simulink model "CDPR_bloques_lazo_abiertoR2020a"  (R2020a)
settings: Solver=ode15s  StartTime=0.0  StopTime=10  MaxStep=0.001  RelTol=1e-30
InitFcn:
  | % The global parameters for simulink are defined by running this script
  | % - Back emf constant           [Kb] (V/rad/sec)
  | % - Motor torque constant       [Kt] (N.m/A)
  | % - Mechanical inertia          [Jm] (kg.m^2)
  | % - Friction coeficient         [Bm] (N.m.s)
  | % - Armature resistance         [Ra] (Ohm)
  | % - Armature inductance         [La] (H)
  | 
  | Kb = 1.25;
  | Kt = 0.516;
  | Jm = 0.0221;
  | Bm = 0.002953;
  | Ra = 2.581;
  | La = 0.0281;
  | b = 0.1;
  | m = 0.5;
  | g = 9.81;
  | r = 0.3;
settings Model: OrderedModelArguments=off  Creator=C20256  LastModifiedBy=C20256
settings DebuggingCC: AlgebraicLoopMsg=none

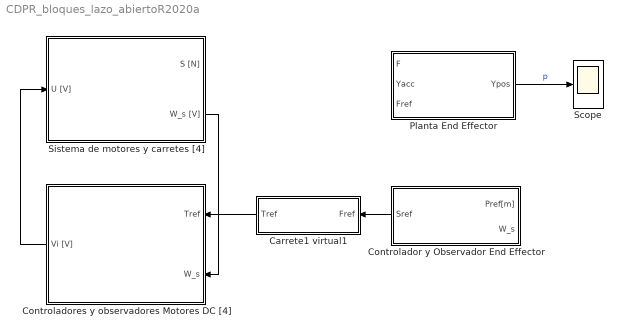
== system CDPR_bloques_lazo_abiertoR2020a ==
  Carrete1 virtual1 : Subsystem
      settings: PortSchema="{\"entries\":[{\"content\":{\"sides\":[{\"content\":{\"connectorIds\":[\"Out1\"]},\"type\":\"ConnectorPlacement.EquallySpacedRectSide\",\"uuid\":\"e435b17b-c2fe-4911-bfed-03351310c969\"},{\"content\":{\"connectorIds\":[\"In1\"],\"side\":\"RIGHT\"},\"type\":\"ConnectorPlacement.EquallySpacedRectSide\",\"uuid\":\"de4daf8e-4374-4970-b69a-ffc749c87b1a\"},{\"content\":{\"connectorIds\":[],\"side\":\"TOP\"},\"type\":\"ConnectorPlacement.EquallySpacedRectSide\",\"uuid\":\"7861d55a-b03c-4daa-b9ee-ff2ad3262c5d\"}]},\"type\":\"ConnectorPlacement.EquallySpacedConnector\",\"uuid\":\"ff68927d-1fa0-407f-8d33-41a83477036e\"}],\"packageUris\":[\"http://schema.mathworks.com/mf0/Connector/19700101\"],\"version\":\"1.0\"}"
  Controlador y Observador End Effector : Subsystem
      settings: PortSchema="{\"entries\":[{\"content\":{\"sides\":[{\"content\":{\"connectorIds\":[\"Out1\"]},\"type\":\"ConnectorPlacement.EquallySpacedRectSide\",\"uuid\":\"e435b17b-c2fe-4911-bfed-03351310c969\"},{\"content\":{\"connectorIds\":[\"In1\",\"In2\"],\"side\":\"RIGHT\"},\"type\":\"ConnectorPlacement.EquallySpacedRectSide\",\"uuid\":\"de4daf8e-4374-4970-b69a-ffc749c87b1a\"},{\"content\":{\"connectorIds\":[],\"side\":\"TOP\"},\"type\":\"ConnectorPlacement.EquallySpacedRectSide\",\"uuid\":\"7861d55a-b03c-4daa-b9ee-ff2ad3262c5d\"}]},\"type\":\"ConnectorPlacement.EquallySpacedConnector\",\"uuid\":\"ff68927d-1fa0-407f-8d33-41a83477036e\"}],\"packageUris\":[\"http://schema.mathworks.com/mf0/Connector/19700101\"],\"version\":\"1.0\"}"
  "Controladores y observadores Motores DC [4] " : Subsystem
  Planta End Effector : Subsystem
      settings: PortSchema="{\"entries\":[{\"content\":{\"sides\":[{\"content\":{\"connectorIds\":[\"In1\",\"Out2\",\"Out3\"]},\"type\":\"ConnectorPlacement.EquallySpacedRectSide\",\"uuid\":\"e435b17b-c2fe-4911-bfed-03351310c969\"},{\"content\":{\"connectorIds\":[\"Out1\"],\"side\":\"RIGHT\"},\"type\":\"ConnectorPlacement.EquallySpacedRectSide\",\"uuid\":\"de4daf8e-4374-4970-b69a-ffc749c87b1a\"},{\"content\":{\"connectorIds\":[],\"side\":\"TOP\"},\"type\":\"ConnectorPlacement.EquallySpacedRectSide\",\"uuid\":\"7861d55a-b03c-4daa-b9ee-ff2ad3262c5d\"}]},\"type\":\"ConnectorPlacement.EquallySpacedConnector\",\"uuid\":\"ff68927d-1fa0-407f-8d33-41a83477036e\"}],\"packageUris\":[\"http://schema.mathworks.com/mf0/Connector/19700101\"],\"version\":\"1.0\"}"
  Scope : Scope
  Sistema de motores y carretes [4] : Subsystem
  wires:
  Planta End Effector/1(Ypos) -> Scope/1  "p"
  "Controladores y observadores Motores DC [4] "/1(Vi [V]) -> Sistema de motores y carretes [4]/1(U [V])
  Sistema de motores y carretes [4]/2(W_s [V]) -> "Controladores y observadores Motores DC [4] "/2(W_s)
  Carrete1 virtual1/1(Tref) -> "Controladores y observadores Motores DC [4] "/1(Tref)
  Controlador y Observador End Effector/1(Sref) -> Carrete1 virtual1/1(Fref)

== system CDPR_bloques_lazo_abiertoR2020a/Carrete1 virtual1 ==
  Fref : Inport
  Gain2 : Gain  Gain=0.05
  Tref : Outport
  wires:
  Fref/1 -> Gain2/1  "Fref"
  Gain2/1 -> Tref/1  "Tref"

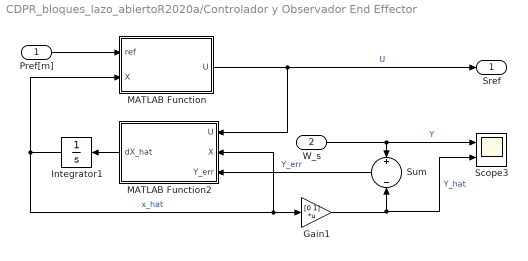
== system CDPR_bloques_lazo_abiertoR2020a/Controlador y Observador End Effector ==
  Pref[m] : Inport
  W_s : Inport  Port=2
  Gain1 : Gain  Gain=[0 1]  Multiplication=Matrix(K*u)
  Integrator1 : Integrator  InitialCondition=[0 0]
  MATLAB Function : MATLAB Function  TreatAsAtomicUnit=on
  MATLAB Function2 : MATLAB Function  TreatAsAtomicUnit=on
  Scope3 : Scope  NumInputPorts=2
  Sum : Sum  Inputs=+||||-
  Sref : Outport
  wires:
  Integrator1/1 -> MATLAB Function/2(X), Gain1/1, MATLAB Function2/2(X)  "x_hat"
  MATLAB Function2/1(dX_hat) -> Integrator1/1
  Sum/1 -> MATLAB Function2/3(Y_err)  "Y_err"
  Pref[m]/1 -> MATLAB Function/1(ref)
  Gain1/1 -> Scope3/2, Sum/2  "Y_hat"
  W_s/1 -> Scope3/1, Sum/1  "Y"
  MATLAB Function/1(U) -> Sref/1, MATLAB Function2/1(U)  "U"

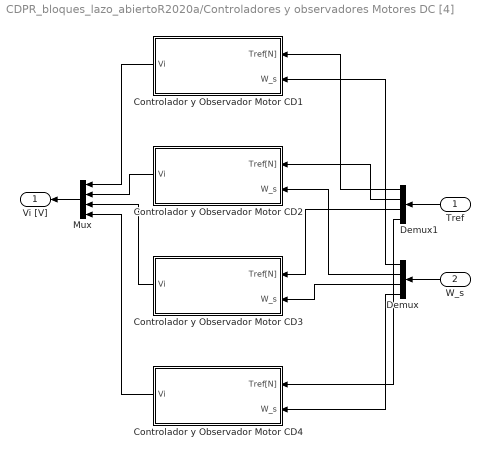
== system CDPR_bloques_lazo_abiertoR2020a/Controladores y observadores Motores DC [4]  ==
  Tref : Inport
  W_s : Inport  Port=2
  Controlador y Observador Motor CD1 : Subsystem
      settings: PortSchema="{\"entries\":[{\"content\":{\"sides\":[{\"content\":{\"connectorIds\":[\"Out1\"]},\"type\":\"ConnectorPlacement.EquallySpacedRectSide\",\"uuid\":\"e435b17b-c2fe-4911-bfed-03351310c969\"},{\"content\":{\"connectorIds\":[\"In1\",\"In2\"],\"side\":\"RIGHT\"},\"type\":\"ConnectorPlacement.EquallySpacedRectSide\",\"uuid\":\"de4daf8e-4374-4970-b69a-ffc749c87b1a\"},{\"content\":{\"connectorIds\":[],\"side\":\"TOP\"},\"type\":\"ConnectorPlacement.EquallySpacedRectSide\",\"uuid\":\"7861d55a-b03c-4daa-b9ee-ff2ad3262c5d\"}]},\"type\":\"ConnectorPlacement.EquallySpacedConnector\",\"uuid\":\"ff68927d-1fa0-407f-8d33-41a83477036e\"}],\"packageUris\":[\"http://schema.mathworks.com/mf0/Connector/19700101\"],\"version\":\"1.0\"}"
  Controlador y Observador Motor CD2 : Subsystem
      settings: PortSchema="{\"entries\":[{\"content\":{\"sides\":[{\"content\":{\"connectorIds\":[\"Out1\"]},\"type\":\"ConnectorPlacement.EquallySpacedRectSide\",\"uuid\":\"e435b17b-c2fe-4911-bfed-03351310c969\"},{\"content\":{\"connectorIds\":[\"In1\",\"In2\"],\"side\":\"RIGHT\"},\"type\":\"ConnectorPlacement.EquallySpacedRectSide\",\"uuid\":\"de4daf8e-4374-4970-b69a-ffc749c87b1a\"},{\"content\":{\"connectorIds\":[],\"side\":\"TOP\"},\"type\":\"ConnectorPlacement.EquallySpacedRectSide\",\"uuid\":\"7861d55a-b03c-4daa-b9ee-ff2ad3262c5d\"}]},\"type\":\"ConnectorPlacement.EquallySpacedConnector\",\"uuid\":\"ff68927d-1fa0-407f-8d33-41a83477036e\"}],\"packageUris\":[\"http://schema.mathworks.com/mf0/Connector/19700101\"],\"version\":\"1.0\"}"
  Controlador y Observador Motor CD3 : Subsystem
      settings: PortSchema="{\"entries\":[{\"content\":{\"sides\":[{\"content\":{\"connectorIds\":[\"Out1\"]},\"type\":\"ConnectorPlacement.EquallySpacedRectSide\",\"uuid\":\"e435b17b-c2fe-4911-bfed-03351310c969\"},{\"content\":{\"connectorIds\":[\"In1\",\"In2\"],\"side\":\"RIGHT\"},\"type\":\"ConnectorPlacement.EquallySpacedRectSide\",\"uuid\":\"de4daf8e-4374-4970-b69a-ffc749c87b1a\"},{\"content\":{\"connectorIds\":[],\"side\":\"TOP\"},\"type\":\"ConnectorPlacement.EquallySpacedRectSide\",\"uuid\":\"7861d55a-b03c-4daa-b9ee-ff2ad3262c5d\"}]},\"type\":\"ConnectorPlacement.EquallySpacedConnector\",\"uuid\":\"ff68927d-1fa0-407f-8d33-41a83477036e\"}],\"packageUris\":[\"http://schema.mathworks.com/mf0/Connector/19700101\"],\"version\":\"1.0\"}"
  Controlador y Observador Motor CD4 : Subsystem
      settings: PortSchema="{\"entries\":[{\"content\":{\"sides\":[{\"content\":{\"connectorIds\":[\"Out1\"]},\"type\":\"ConnectorPlacement.EquallySpacedRectSide\",\"uuid\":\"e435b17b-c2fe-4911-bfed-03351310c969\"},{\"content\":{\"connectorIds\":[\"In1\",\"In2\"],\"side\":\"RIGHT\"},\"type\":\"ConnectorPlacement.EquallySpacedRectSide\",\"uuid\":\"de4daf8e-4374-4970-b69a-ffc749c87b1a\"},{\"content\":{\"connectorIds\":[],\"side\":\"TOP\"},\"type\":\"ConnectorPlacement.EquallySpacedRectSide\",\"uuid\":\"7861d55a-b03c-4daa-b9ee-ff2ad3262c5d\"}]},\"type\":\"ConnectorPlacement.EquallySpacedConnector\",\"uuid\":\"ff68927d-1fa0-407f-8d33-41a83477036e\"}],\"packageUris\":[\"http://schema.mathworks.com/mf0/Connector/19700101\"],\"version\":\"1.0\"}"
  Demux : Demux
  Demux1 : Demux
  Mux : Mux
  Vi [V] : Outport
  wires:
  W_s/1 -> Demux/1
  Tref/1 -> Demux1/1
  Demux1/1 -> Controlador y Observador Motor CD1/1(Tref[N])
  Demux1/2 -> Controlador y Observador Motor CD2/1(Tref[N])
  Demux1/3 -> Controlador y Observador Motor CD3/1(Tref[N])
  Demux1/4 -> Controlador y Observador Motor CD4/1(Tref[N])
  Demux/1 -> Controlador y Observador Motor CD1/2(W_s)
  Demux/2 -> Controlador y Observador Motor CD2/2(W_s)
  Demux/3 -> Controlador y Observador Motor CD3/2(W_s)
  Demux/4 -> Controlador y Observador Motor CD4/2(W_s)
  Controlador y Observador Motor CD4/1(Vi) -> Mux/4
  Controlador y Observador Motor CD3/1(Vi) -> Mux/3
  Mux/1 -> Vi [V]/1
  Controlador y Observador Motor CD2/1(Vi) -> Mux/2
  Controlador y Observador Motor CD1/1(Vi) -> Mux/1

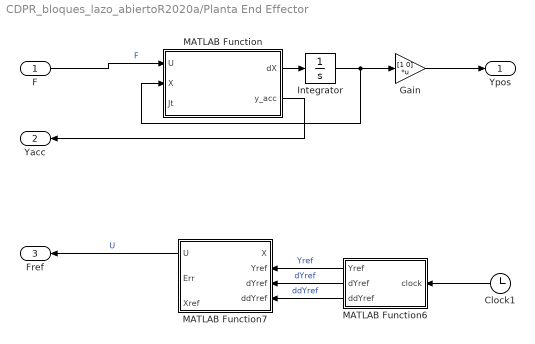
== system CDPR_bloques_lazo_abiertoR2020a/Planta End Effector ==
  F : Inport
  Clock1 : Clock
  Gain : Gain  Gain=[1 0]  Multiplication=Matrix(K*u)
  Integrator : Integrator  InitialCondition=[0 0]
  MATLAB Function : MATLAB Function  TreatAsAtomicUnit=on
  MATLAB Function6 : MATLAB Function  TreatAsAtomicUnit=on
  MATLAB Function7 : MATLAB Function  TreatAsAtomicUnit=on
  Ypos : Outport
  Yacc : Outport  Port=2
  Fref : Outport  Port=3
  wires:
  Integrator/1 -> Gain/1, MATLAB Function/2(X)
  MATLAB Function/1(dX) -> Integrator/1
  Gain/1 -> Ypos/1
  MATLAB Function/2(y_acc) -> Yacc/1
  Clock1/1 -> MATLAB Function6/1(clock)
  MATLAB Function6/1(Yref) -> MATLAB Function7/2(Yref)  "Yref"
  MATLAB Function6/2(dYref) -> MATLAB Function7/3(dYref)  "dYref"
  MATLAB Function6/3(ddYref) -> MATLAB Function7/4(ddYref)  "ddYref"
  MATLAB Function7/1(U) -> Fref/1  "U"
  F/1 -> MATLAB Function/1(U)  "F"

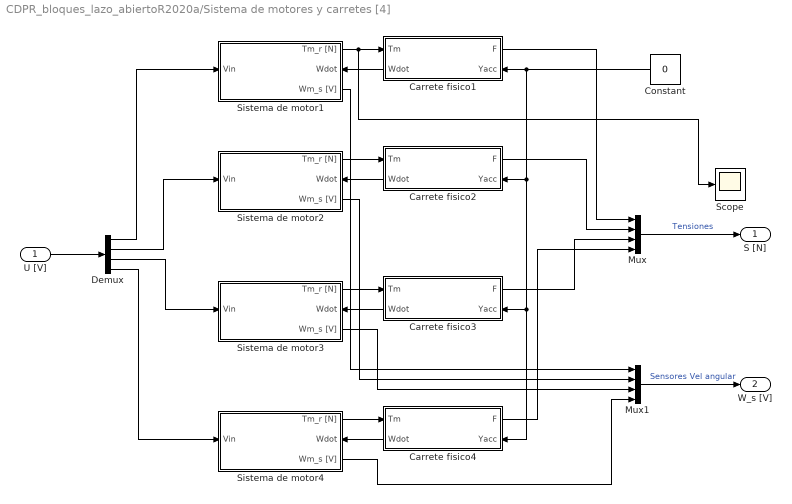
== system CDPR_bloques_lazo_abiertoR2020a/Sistema de motores y carretes [4] ==
  U [V] : Inport
  Carrete fisico1 : Subsystem
      settings: PortSchema="{\"entries\":[{\"content\":{\"sides\":[{\"content\":{\"connectorIds\":[\"In1\",\"Out2\"]},\"type\":\"ConnectorPlacement.EquallySpacedRectSide\",\"uuid\":\"e435b17b-c2fe-4911-bfed-03351310c969\"},{\"content\":{\"connectorIds\":[\"Out1\",\"In2\"],\"side\":\"RIGHT\"},\"type\":\"ConnectorPlacement.EquallySpacedRectSide\",\"uuid\":\"de4daf8e-4374-4970-b69a-ffc749c87b1a\"},{\"content\":{\"connectorIds\":[],\"side\":\"TOP\"},\"type\":\"ConnectorPlacement.EquallySpacedRectSide\",\"uuid\":\"7861d55a-b03c-4daa-b9ee-ff2ad3262c5d\"}]},\"type\":\"ConnectorPlacement.EquallySpacedConnector\",\"uuid\":\"ff68927d-1fa0-407f-8d33-41a83477036e\"}],\"packageUris\":[\"http://schema.mathworks.com/mf0/Connector/19700101\"],\"version\":\"1.0\"}"
  Carrete fisico2 : Subsystem
      settings: PortSchema="{\"entries\":[{\"content\":{\"sides\":[{\"content\":{\"connectorIds\":[\"In1\",\"Out2\"]},\"type\":\"ConnectorPlacement.EquallySpacedRectSide\",\"uuid\":\"e435b17b-c2fe-4911-bfed-03351310c969\"},{\"content\":{\"connectorIds\":[\"Out1\",\"In2\"],\"side\":\"RIGHT\"},\"type\":\"ConnectorPlacement.EquallySpacedRectSide\",\"uuid\":\"de4daf8e-4374-4970-b69a-ffc749c87b1a\"},{\"content\":{\"connectorIds\":[],\"side\":\"TOP\"},\"type\":\"ConnectorPlacement.EquallySpacedRectSide\",\"uuid\":\"7861d55a-b03c-4daa-b9ee-ff2ad3262c5d\"}]},\"type\":\"ConnectorPlacement.EquallySpacedConnector\",\"uuid\":\"ff68927d-1fa0-407f-8d33-41a83477036e\"}],\"packageUris\":[\"http://schema.mathworks.com/mf0/Connector/19700101\"],\"version\":\"1.0\"}"
  Carrete fisico3 : Subsystem
      settings: PortSchema="{\"entries\":[{\"content\":{\"sides\":[{\"content\":{\"connectorIds\":[\"In1\",\"Out2\"]},\"type\":\"ConnectorPlacement.EquallySpacedRectSide\",\"uuid\":\"e435b17b-c2fe-4911-bfed-03351310c969\"},{\"content\":{\"connectorIds\":[\"Out1\",\"In2\"],\"side\":\"RIGHT\"},\"type\":\"ConnectorPlacement.EquallySpacedRectSide\",\"uuid\":\"de4daf8e-4374-4970-b69a-ffc749c87b1a\"},{\"content\":{\"connectorIds\":[],\"side\":\"TOP\"},\"type\":\"ConnectorPlacement.EquallySpacedRectSide\",\"uuid\":\"7861d55a-b03c-4daa-b9ee-ff2ad3262c5d\"}]},\"type\":\"ConnectorPlacement.EquallySpacedConnector\",\"uuid\":\"ff68927d-1fa0-407f-8d33-41a83477036e\"}],\"packageUris\":[\"http://schema.mathworks.com/mf0/Connector/19700101\"],\"version\":\"1.0\"}"
  Carrete fisico4 : Subsystem
      settings: PortSchema="{\"entries\":[{\"content\":{\"sides\":[{\"content\":{\"connectorIds\":[\"In1\",\"Out2\"]},\"type\":\"ConnectorPlacement.EquallySpacedRectSide\",\"uuid\":\"e435b17b-c2fe-4911-bfed-03351310c969\"},{\"content\":{\"connectorIds\":[\"Out1\",\"In2\"],\"side\":\"RIGHT\"},\"type\":\"ConnectorPlacement.EquallySpacedRectSide\",\"uuid\":\"de4daf8e-4374-4970-b69a-ffc749c87b1a\"},{\"content\":{\"connectorIds\":[],\"side\":\"TOP\"},\"type\":\"ConnectorPlacement.EquallySpacedRectSide\",\"uuid\":\"7861d55a-b03c-4daa-b9ee-ff2ad3262c5d\"}]},\"type\":\"ConnectorPlacement.EquallySpacedConnector\",\"uuid\":\"ff68927d-1fa0-407f-8d33-41a83477036e\"}],\"packageUris\":[\"http://schema.mathworks.com/mf0/Connector/19700101\"],\"version\":\"1.0\"}"
  Constant : Constant  Value=0
  Demux : Demux
  Mux : Mux
  Mux1 : Mux
  Scope : Scope
  Sistema de motor1 : Subsystem
      settings: PortSchema="{\"entries\":[{\"content\":{\"sides\":[{\"content\":{\"connectorIds\":[\"In1\"]},\"type\":\"ConnectorPlacement.EquallySpacedRectSide\",\"uuid\":\"e435b17b-c2fe-4911-bfed-03351310c969\"},{\"content\":{\"connectorIds\":[\"Out1\",\"In2\",\"Out2\"],\"side\":\"RIGHT\"},\"type\":\"ConnectorPlacement.EquallySpacedRectSide\",\"uuid\":\"de4daf8e-4374-4970-b69a-ffc749c87b1a\"},{\"content\":{\"connectorIds\":[],\"side\":\"TOP\"},\"type\":\"ConnectorPlacement.EquallySpacedRectSide\",\"uuid\":\"7861d55a-b03c-4daa-b9ee-ff2ad3262c5d\"}]},\"type\":\"ConnectorPlacement.EquallySpacedConnector\",\"uuid\":\"ff68927d-1fa0-407f-8d33-41a83477036e\"}],\"packageUris\":[\"http://schema.mathworks.com/mf0/Connector/19700101\"],\"version\":\"1.0\"}"
  Sistema de motor2 : Subsystem
      settings: PortSchema="{\"entries\":[{\"content\":{\"sides\":[{\"content\":{\"connectorIds\":[\"In1\"]},\"type\":\"ConnectorPlacement.EquallySpacedRectSide\",\"uuid\":\"e435b17b-c2fe-4911-bfed-03351310c969\"},{\"content\":{\"connectorIds\":[\"Out1\",\"In2\",\"Out2\"],\"side\":\"RIGHT\"},\"type\":\"ConnectorPlacement.EquallySpacedRectSide\",\"uuid\":\"de4daf8e-4374-4970-b69a-ffc749c87b1a\"},{\"content\":{\"connectorIds\":[],\"side\":\"TOP\"},\"type\":\"ConnectorPlacement.EquallySpacedRectSide\",\"uuid\":\"7861d55a-b03c-4daa-b9ee-ff2ad3262c5d\"}]},\"type\":\"ConnectorPlacement.EquallySpacedConnector\",\"uuid\":\"ff68927d-1fa0-407f-8d33-41a83477036e\"}],\"packageUris\":[\"http://schema.mathworks.com/mf0/Connector/19700101\"],\"version\":\"1.0\"}"
  Sistema de motor3 : Subsystem
      settings: PortSchema="{\"entries\":[{\"content\":{\"sides\":[{\"content\":{\"connectorIds\":[\"In1\"]},\"type\":\"ConnectorPlacement.EquallySpacedRectSide\",\"uuid\":\"e435b17b-c2fe-4911-bfed-03351310c969\"},{\"content\":{\"connectorIds\":[\"Out1\",\"In2\",\"Out2\"],\"side\":\"RIGHT\"},\"type\":\"ConnectorPlacement.EquallySpacedRectSide\",\"uuid\":\"de4daf8e-4374-4970-b69a-ffc749c87b1a\"},{\"content\":{\"connectorIds\":[],\"side\":\"TOP\"},\"type\":\"ConnectorPlacement.EquallySpacedRectSide\",\"uuid\":\"7861d55a-b03c-4daa-b9ee-ff2ad3262c5d\"}]},\"type\":\"ConnectorPlacement.EquallySpacedConnector\",\"uuid\":\"ff68927d-1fa0-407f-8d33-41a83477036e\"}],\"packageUris\":[\"http://schema.mathworks.com/mf0/Connector/19700101\"],\"version\":\"1.0\"}"
  Sistema de motor4 : Subsystem
      settings: PortSchema="{\"entries\":[{\"content\":{\"sides\":[{\"content\":{\"connectorIds\":[\"In1\"]},\"type\":\"ConnectorPlacement.EquallySpacedRectSide\",\"uuid\":\"e435b17b-c2fe-4911-bfed-03351310c969\"},{\"content\":{\"connectorIds\":[\"Out1\",\"In2\",\"Out2\"],\"side\":\"RIGHT\"},\"type\":\"ConnectorPlacement.EquallySpacedRectSide\",\"uuid\":\"de4daf8e-4374-4970-b69a-ffc749c87b1a\"},{\"content\":{\"connectorIds\":[],\"side\":\"TOP\"},\"type\":\"ConnectorPlacement.EquallySpacedRectSide\",\"uuid\":\"7861d55a-b03c-4daa-b9ee-ff2ad3262c5d\"}]},\"type\":\"ConnectorPlacement.EquallySpacedConnector\",\"uuid\":\"ff68927d-1fa0-407f-8d33-41a83477036e\"}],\"packageUris\":[\"http://schema.mathworks.com/mf0/Connector/19700101\"],\"version\":\"1.0\"}"
  S [N] : Outport
  W_s [V] : Outport  Port=2
  wires:
  Sistema de motor3/2(Wm_s [V]) -> Mux1/3
  Carrete fisico3/2(Wdot) -> Sistema de motor3/2(Wdot)
  Sistema de motor1/2(Wm_s [V]) -> Mux1/1
  Carrete fisico2/2(Wdot) -> Sistema de motor2/2(Wdot)
  Sistema de motor3/1(Tm_r [N]) -> Carrete fisico3/1(Tm)
  Sistema de motor4/2(Wm_s [V]) -> Mux1/4
  Sistema de motor1/1(Tm_r [N]) -> Scope/1, Carrete fisico1/1(Tm)
  Sistema de motor2/2(Wm_s [V]) -> Mux1/2
  Carrete fisico4/2(Wdot) -> Sistema de motor4/2(Wdot)
  Sistema de motor2/1(Tm_r [N]) -> Carrete fisico2/1(Tm)
  Carrete fisico1/2(Wdot) -> Sistema de motor1/2(Wdot)
  Sistema de motor4/1(Tm_r [N]) -> Carrete fisico4/1(Tm)
  Demux/1 -> Sistema de motor1/1(Vin)
  Demux/2 -> Sistema de motor2/1(Vin)
  Demux/3 -> Sistema de motor3/1(Vin)
  Demux/4 -> Sistema de motor4/1(Vin)
  U [V]/1 -> Demux/1
  Carrete fisico2/1(F) -> Mux/2
  Carrete fisico1/1(F) -> Mux/1
  Carrete fisico3/1(F) -> Mux/3
  Carrete fisico4/1(F) -> Mux/4
  Mux1/1 -> W_s [V]/1  "Sensores Vel angular"
  Mux/1 -> S [N]/1  "Tensiones"
  Constant/1 -> Carrete fisico4/2(Yacc), Carrete fisico3/2(Yacc), Carrete fisico2/2(Yacc), Carrete fisico1/2(Yacc)

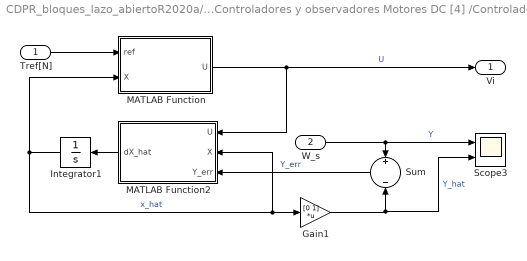
== system CDPR_bloques_lazo_abiertoR2020a/Controladores y observadores Motores DC [4] /Controlador y Observador Motor CD1 ==
  Tref[N] : Inport
  W_s : Inport  Port=2
  Gain1 : Gain  Gain=[0 1]  Multiplication=Matrix(K*u)
  Integrator1 : Integrator  InitialCondition=[0 0]
  MATLAB Function : MATLAB Function  TreatAsAtomicUnit=on
  MATLAB Function2 : MATLAB Function  TreatAsAtomicUnit=on
  Scope3 : Scope  NumInputPorts=2
  Sum : Sum  Inputs=+||||-
  Vi : Outport
  wires:
  Integrator1/1 -> MATLAB Function/2(X), Gain1/1, MATLAB Function2/2(X)  "x_hat"
  MATLAB Function2/1(dX_hat) -> Integrator1/1
  Sum/1 -> MATLAB Function2/3(Y_err)  "Y_err"
  Tref[N]/1 -> MATLAB Function/1(ref)
  Gain1/1 -> Scope3/2, Sum/2  "Y_hat"
  W_s/1 -> Scope3/1, Sum/1  "Y"
  MATLAB Function/1(U) -> Vi/1, MATLAB Function2/1(U)  "U"

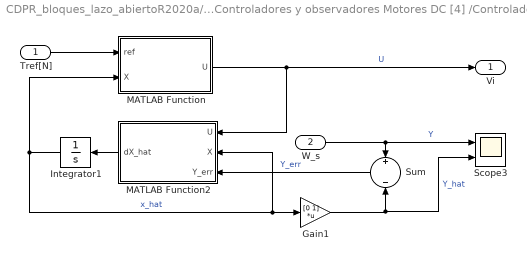
== system CDPR_bloques_lazo_abiertoR2020a/Controladores y observadores Motores DC [4] /Controlador y Observador Motor CD2 ==
  Tref[N] : Inport
  W_s : Inport  Port=2
  Gain1 : Gain  Gain=[0 1]  Multiplication=Matrix(K*u)
  Integrator1 : Integrator  InitialCondition=[0 0]
  MATLAB Function : MATLAB Function  TreatAsAtomicUnit=on
  MATLAB Function2 : MATLAB Function  TreatAsAtomicUnit=on
  Scope3 : Scope  NumInputPorts=2
  Sum : Sum  Inputs=+||||-
  Vi : Outport
  wires:
  Integrator1/1 -> MATLAB Function/2(X), Gain1/1, MATLAB Function2/2(X)  "x_hat"
  MATLAB Function2/1(dX_hat) -> Integrator1/1
  Sum/1 -> MATLAB Function2/3(Y_err)  "Y_err"
  Tref[N]/1 -> MATLAB Function/1(ref)
  Gain1/1 -> Scope3/2, Sum/2  "Y_hat"
  W_s/1 -> Scope3/1, Sum/1  "Y"
  MATLAB Function/1(U) -> Vi/1, MATLAB Function2/1(U)  "U"

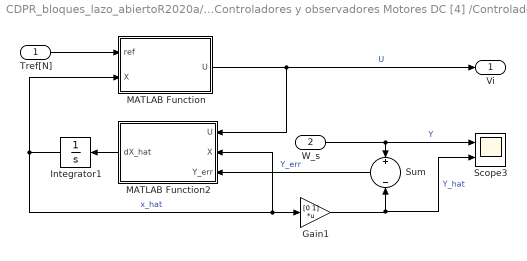
== system CDPR_bloques_lazo_abiertoR2020a/Controladores y observadores Motores DC [4] /Controlador y Observador Motor CD3 ==
  Tref[N] : Inport
  W_s : Inport  Port=2
  Gain1 : Gain  Gain=[0 1]  Multiplication=Matrix(K*u)
  Integrator1 : Integrator  InitialCondition=[0 0]
  MATLAB Function : MATLAB Function  TreatAsAtomicUnit=on
  MATLAB Function2 : MATLAB Function  TreatAsAtomicUnit=on
  Scope3 : Scope  NumInputPorts=2
  Sum : Sum  Inputs=+||||-
  Vi : Outport
  wires:
  Integrator1/1 -> MATLAB Function/2(X), Gain1/1, MATLAB Function2/2(X)  "x_hat"
  MATLAB Function2/1(dX_hat) -> Integrator1/1
  Sum/1 -> MATLAB Function2/3(Y_err)  "Y_err"
  Tref[N]/1 -> MATLAB Function/1(ref)
  Gain1/1 -> Scope3/2, Sum/2  "Y_hat"
  W_s/1 -> Scope3/1, Sum/1  "Y"
  MATLAB Function/1(U) -> Vi/1, MATLAB Function2/1(U)  "U"

== system CDPR_bloques_lazo_abiertoR2020a/Controladores y observadores Motores DC [4] /Controlador y Observador Motor CD4 ==
  Tref[N] : Inport
  W_s : Inport  Port=2
  Gain1 : Gain  Gain=[0 1]  Multiplication=Matrix(K*u)
  Integrator1 : Integrator  InitialCondition=[0 0]
  MATLAB Function : MATLAB Function  TreatAsAtomicUnit=on
  MATLAB Function2 : MATLAB Function  TreatAsAtomicUnit=on
  Scope3 : Scope  NumInputPorts=2
  Sum : Sum  Inputs=+||||-
  Vi : Outport
  wires:
  Integrator1/1 -> MATLAB Function/2(X), Gain1/1, MATLAB Function2/2(X)  "x_hat"
  MATLAB Function2/1(dX_hat) -> Integrator1/1
  Sum/1 -> MATLAB Function2/3(Y_err)  "Y_err"
  Tref[N]/1 -> MATLAB Function/1(ref)
  Gain1/1 -> Scope3/2, Sum/2  "Y_hat"
  W_s/1 -> Scope3/1, Sum/1  "Y"
  MATLAB Function/1(U) -> Vi/1, MATLAB Function2/1(U)  "U"

== system CDPR_bloques_lazo_abiertoR2020a/Sistema de motores y carretes [4]/Carrete fisico1 ==
  Tm : Inport
  Yacc : Inport  Port=2
  Gain : Gain  Gain=1/0.05
  Gain1 : Gain  Gain=1/0.05
  F : Outport
  Wdot : Outport  Port=2
  wires:
  Tm/1 -> Gain/1  "Tm"
  Gain/1 -> F/1  "F"
  Yacc/1 -> Gain1/1  "Yacc"
  Gain1/1 -> Wdot/1  "Acc ang"

== system CDPR_bloques_lazo_abiertoR2020a/Sistema de motores y carretes [4]/Carrete fisico2 ==
  Tm : Inport
  Yacc : Inport  Port=2
  Gain : Gain  Gain=1/0.05
  Gain1 : Gain  Gain=1/0.05
  F : Outport
  Wdot : Outport  Port=2
  wires:
  Tm/1 -> Gain/1  "Tm"
  Gain/1 -> F/1  "F"
  Yacc/1 -> Gain1/1  "Yacc"
  Gain1/1 -> Wdot/1  "Acc ang"

== system CDPR_bloques_lazo_abiertoR2020a/Sistema de motores y carretes [4]/Carrete fisico3 ==
  Tm : Inport
  Yacc : Inport  Port=2
  Gain : Gain  Gain=1/0.05
  Gain1 : Gain  Gain=1/0.05
  F : Outport
  Wdot : Outport  Port=2
  wires:
  Tm/1 -> Gain/1  "Tm"
  Gain/1 -> F/1  "F"
  Yacc/1 -> Gain1/1  "Yacc"
  Gain1/1 -> Wdot/1  "Acc ang"

== system CDPR_bloques_lazo_abiertoR2020a/Sistema de motores y carretes [4]/Carrete fisico4 ==
  Tm : Inport
  Yacc : Inport  Port=2
  Gain : Gain  Gain=1/0.05
  Gain1 : Gain  Gain=1/0.05
  F : Outport
  Wdot : Outport  Port=2
  wires:
  Tm/1 -> Gain/1  "Tm"
  Gain/1 -> F/1  "F"
  Yacc/1 -> Gain1/1  "Yacc"
  Gain1/1 -> Wdot/1  "Acc ang"

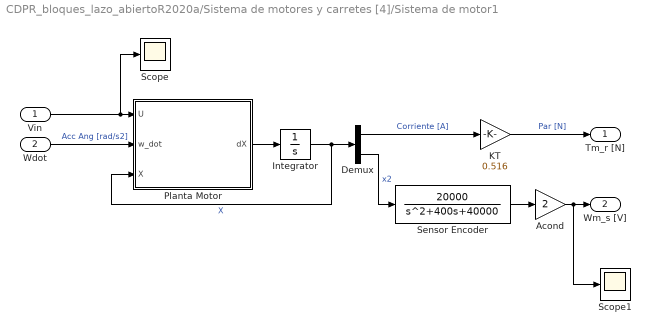
== system CDPR_bloques_lazo_abiertoR2020a/Sistema de motores y carretes [4]/Sistema de motor1 ==
  Vin : Inport
  Wdot : Inport  Port=2
  Acond : Gain  Gain=2
  Demux : Demux  Outputs=2
  Integrator : Integrator  InitialCondition=[0 0]
  KT : Gain  Gain=0.516
  Planta Motor : MATLAB Function  TreatAsAtomicUnit=on
  Scope : Scope
  Scope1 : Scope
  Sensor Encoder : TransferFcn  Numerator=[20000]  Denominator=[1 400 40000]
  Tm_r [N] : Outport
  Wm_s [V] : Outport  Port=2
  wires:
  Planta Motor/1(dX) -> Integrator/1
  Integrator/1 -> Planta Motor/3(X), Demux/1  "X"
  KT/1 -> Tm_r [N]/1  "Par [N]"
  Demux/1 -> KT/1  "Corriente [A]"
  Acond/1 -> Scope1/1, Wm_s [V]/1
  Sensor Encoder/1 -> Acond/1
  Demux/2 -> Sensor Encoder/1  "x2"
  Wdot/1 -> Planta Motor/2(w_dot)  "Acc Ang [rad/s2]"
  Vin/1 -> Scope/1, Planta Motor/1(U)

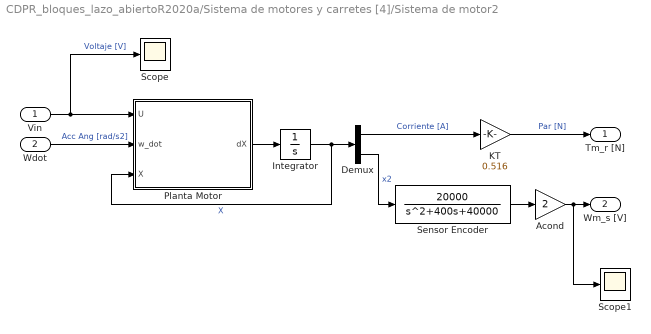
== system CDPR_bloques_lazo_abiertoR2020a/Sistema de motores y carretes [4]/Sistema de motor2 ==
  Vin : Inport
  Wdot : Inport  Port=2
  Acond : Gain  Gain=2
  Demux : Demux  Outputs=2
  Integrator : Integrator  InitialCondition=[0 0]
  KT : Gain  Gain=0.516
  Planta Motor : MATLAB Function  TreatAsAtomicUnit=on
  Scope : Scope
  Scope1 : Scope
  Sensor Encoder : TransferFcn  Numerator=[20000]  Denominator=[1 400 40000]
  Tm_r [N] : Outport
  Wm_s [V] : Outport  Port=2
  wires:
  Planta Motor/1(dX) -> Integrator/1
  Integrator/1 -> Planta Motor/3(X), Demux/1  "X"
  KT/1 -> Tm_r [N]/1  "Par [N]"
  Demux/1 -> KT/1  "Corriente [A]"
  Wdot/1 -> Planta Motor/2(w_dot)  "Acc Ang [rad/s2]"
  Vin/1 -> Scope/1, Planta Motor/1(U)  "Voltaje [V]"
  Acond/1 -> Scope1/1, Wm_s [V]/1
  Sensor Encoder/1 -> Acond/1
  Demux/2 -> Sensor Encoder/1  "x2"

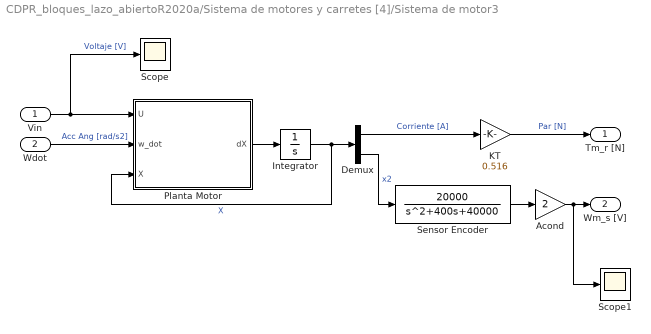
== system CDPR_bloques_lazo_abiertoR2020a/Sistema de motores y carretes [4]/Sistema de motor3 ==
  Vin : Inport
  Wdot : Inport  Port=2
  Acond : Gain  Gain=2
  Demux : Demux  Outputs=2
  Integrator : Integrator  InitialCondition=[0 0]
  KT : Gain  Gain=0.516
  Planta Motor : MATLAB Function  TreatAsAtomicUnit=on
  Scope : Scope
  Scope1 : Scope
  Sensor Encoder : TransferFcn  Numerator=[20000]  Denominator=[1 400 40000]
  Tm_r [N] : Outport
  Wm_s [V] : Outport  Port=2
  wires:
  Planta Motor/1(dX) -> Integrator/1
  Integrator/1 -> Planta Motor/3(X), Demux/1  "X"
  KT/1 -> Tm_r [N]/1  "Par [N]"
  Demux/1 -> KT/1  "Corriente [A]"
  Wdot/1 -> Planta Motor/2(w_dot)  "Acc Ang [rad/s2]"
  Vin/1 -> Scope/1, Planta Motor/1(U)  "Voltaje [V]"
  Acond/1 -> Scope1/1, Wm_s [V]/1
  Sensor Encoder/1 -> Acond/1
  Demux/2 -> Sensor Encoder/1  "x2"

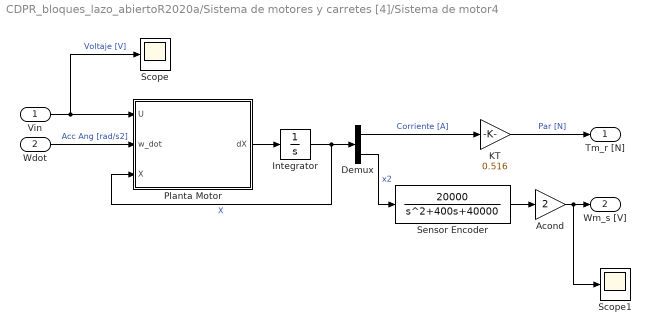
== system CDPR_bloques_lazo_abiertoR2020a/Sistema de motores y carretes [4]/Sistema de motor4 ==
  Vin : Inport
  Wdot : Inport  Port=2
  Acond : Gain  Gain=2
  Demux : Demux  Outputs=2
  Integrator : Integrator  InitialCondition=[0 0]
  KT : Gain  Gain=0.516
  Planta Motor : MATLAB Function  TreatAsAtomicUnit=on
  Scope : Scope
  Scope1 : Scope
  Sensor Encoder : TransferFcn  Numerator=[20000]  Denominator=[1 400 40000]
  Tm_r [N] : Outport
  Wm_s [V] : Outport  Port=2
  wires:
  Planta Motor/1(dX) -> Integrator/1
  Integrator/1 -> Planta Motor/3(X), Demux/1  "X"
  KT/1 -> Tm_r [N]/1  "Par [N]"
  Demux/1 -> KT/1  "Corriente [A]"
  Wdot/1 -> Planta Motor/2(w_dot)  "Acc Ang [rad/s2]"
  Vin/1 -> Scope/1, Planta Motor/1(U)  "Voltaje [V]"
  Acond/1 -> Scope1/1, Wm_s [V]/1
  Sensor Encoder/1 -> Acond/1
  Demux/2 -> Sensor Encoder/1  "x2"

== matlab function CDPR_bloques_lazo_abiertoR2020a/Sistema de motores y carretes [4]/Sistema de motor4/Planta Motor ==
  data: U input; w_dot input; dX output; X input
function dX  = MotorCD(U, w_dot, X)
%Parametros del sistema

Kb = 1.25;
Kt = 0.516;
Jm = 0.0221;
Bm = 0.002953;
Ra = 2.581;
La = 0.0281;

a11 = -Ra/La;
a12 = -Kb/La;
a21 =  Kt/Jm;
a22 = -Bm/Jm;
b11 = 1/La;
b22 = 0;
f11 = 0;
f22 = -1/Jm;
 
A = [a11 a12; a21 a22]; 
B = [b11; b22];

F = [f11; f22];
TL = -Kt * X(1) + Jm * w_dot + Bm * X(2) ;
 
dX = A*X + B*U + F*TL;
end

== matlab function CDPR_bloques_lazo_abiertoR2020a/Controladores y observadores Motores DC [4] /Controlador y Observador Motor CD2/MATLAB Function ==
  settings: updateMethod=CONTINUOUS
  data: ref input; X input; U output
function U  = Controlador(ref, X)
Kb = 1.25;
Kt = 0.516;
Jm = 0.0221;
Bm = 0.002953;
Ra = 2.581;
La = 0.0281;

a11 = -Ra/La;
a12 = -Kb/La;
a21 =  Kt/Jm;
a22 = -Bm/Jm;
b11 = 1/La;
b22 = 0;
 
A = [a11 a12; a21 a22]; 
B = [b11; b22];
C = [Kt 0];
Pd = [-4 -4];
%Controlador
Mc = [B A*B]
H = (A-Pd(1)*eye(2))*(A-Pd(2)*eye(2));
K = -[0 1] * inv(Mc) * H;
F = 1/(C*inv(-A-B*K) * B);

U = K*X + F*ref;
end

== matlab function CDPR_bloques_lazo_abiertoR2020a/Controladores y observadores Motores DC [4] /Controlador y Observador Motor CD2/MATLAB Function2 ==
  data: U input; X input; Y_err input; dX_hat output
function dX_hat = Observador(U, X, Y_err)
Kb = 1.25;
Kt = 0.516;
Jm = 0.0221;
Bm = 0.002953;
Ra = 2.581;
La = 0.0281;

a11 = -Ra/La;
a12 = -Kb/La;
a21 =  Kt/Jm;
a22 = -Bm/Jm;
b11 = 1/La;
b22 = 0;
 
A = [a11 a12; a21 a22]; 
B = [b11; b22];
C = [0 1];

Pdo = [-80 -80];

Mo1 = [C ;
      C*A];
Ho = (A-Pdo(1)*eye(2))*(A-Pdo(2)*eye(2));
L = -Ho * inv(Mo1) * [0 1].';
%Espacio de estados
dX_hat = A*X + B*U - L*Y_err;
end

== matlab function CDPR_bloques_lazo_abiertoR2020a/Controladores y observadores Motores DC [4] /Controlador y Observador Motor CD3/MATLAB Function ==
  settings: updateMethod=CONTINUOUS
  data: ref input; X input; U output
function U  = Controlador(ref, X)
Kb = 1.25;
Kt = 0.516;
Jm = 0.0221;
Bm = 0.002953;
Ra = 2.581;
La = 0.0281;

a11 = -Ra/La;
a12 = -Kb/La;
a21 =  Kt/Jm;
a22 = -Bm/Jm;
b11 = 1/La;
b22 = 0;
 
A = [a11 a12; a21 a22]; 
B = [b11; b22];
C = [Kt 0];
Pd = [-4 -4];
%Controlador
Mc = [B A*B]
H = (A-Pd(1)*eye(2))*(A-Pd(2)*eye(2));
K = -[0 1] * inv(Mc) * H;
F = 1/(C*inv(-A-B*K) * B);

U = K*X + F*ref;
end

== matlab function CDPR_bloques_lazo_abiertoR2020a/Controladores y observadores Motores DC [4] /Controlador y Observador Motor CD3/MATLAB Function2 ==
  data: U input; X input; Y_err input; dX_hat output
function dX_hat = Observador(U, X, Y_err)
Kb = 1.25;
Kt = 0.516;
Jm = 0.0221;
Bm = 0.002953;
Ra = 2.581;
La = 0.0281;

a11 = -Ra/La;
a12 = -Kb/La;
a21 =  Kt/Jm;
a22 = -Bm/Jm;
b11 = 1/La;
b22 = 0;
 
A = [a11 a12; a21 a22]; 
B = [b11; b22];
C = [0 1];

Pdo = [-80 -80];

Mo1 = [C ;
      C*A];
Ho = (A-Pdo(1)*eye(2))*(A-Pdo(2)*eye(2));
L = -Ho * inv(Mo1) * [0 1].';
%Espacio de estados
dX_hat = A*X + B*U - L*Y_err;
end

== matlab function CDPR_bloques_lazo_abiertoR2020a/Controladores y observadores Motores DC [4] /Controlador y Observador Motor CD4/MATLAB Function ==
  settings: updateMethod=CONTINUOUS
  data: ref input; X input; U output
function U  = Controlador(ref, X)
Kb = 1.25;
Kt = 0.516;
Jm = 0.0221;
Bm = 0.002953;
Ra = 2.581;
La = 0.0281;

a11 = -Ra/La;
a12 = -Kb/La;
a21 =  Kt/Jm;
a22 = -Bm/Jm;
b11 = 1/La;
b22 = 0;
 
A = [a11 a12; a21 a22]; 
B = [b11; b22];
C = [Kt 0];
Pd = [-4 -4];
%Controlador
Mc = [B A*B]
H = (A-Pd(1)*eye(2))*(A-Pd(2)*eye(2));
K = -[0 1] * inv(Mc) * H;
F = 1/(C*inv(-A-B*K) * B);

U = K*X + F*ref;
end

== matlab function CDPR_bloques_lazo_abiertoR2020a/Controladores y observadores Motores DC [4] /Controlador y Observador Motor CD4/MATLAB Function2 ==
  data: U input; X input; Y_err input; dX_hat output
function dX_hat = Observador(U, X, Y_err)
Kb = 1.25;
Kt = 0.516;
Jm = 0.0221;
Bm = 0.002953;
Ra = 2.581;
La = 0.0281;

a11 = -Ra/La;
a12 = -Kb/La;
a21 =  Kt/Jm;
a22 = -Bm/Jm;
b11 = 1/La;
b22 = 0;
 
A = [a11 a12; a21 a22]; 
B = [b11; b22];
C = [0 1];

Pdo = [-80 -80];

Mo1 = [C ;
      C*A];
Ho = (A-Pdo(1)*eye(2))*(A-Pdo(2)*eye(2));
L = -Ho * inv(Mo1) * [0 1].';
%Espacio de estados
dX_hat = A*X + B*U - L*Y_err;
end

== matlab function CDPR_bloques_lazo_abiertoR2020a/Controlador y Observador End Effector/MATLAB Function ==
  settings: updateMethod=CONTINUOUS
  data: ref input; X input; U output
function U  = Controlador(ref, X)
Kb = 1.25;
Kt = 0.516;
Jm = 0.0221;
Bm = 0.002953;
Ra = 2.581;
La = 0.0281;

a11 = -Ra/La;
a12 = -Kb/La;
a21 =  Kt/Jm;
a22 = -Bm/Jm;
b11 = 1/La;
b22 = 0;
 
A = [a11 a12; a21 a22]; 
B = [b11; b22];
C = [Kt 0];
Pd = [-4 -4];
%Controlador
Mc = [B A*B]
H = (A-Pd(1)*eye(2))*(A-Pd(2)*eye(2));
K = -[0 1] * inv(Mc) * H;
F = 1/(C*inv(-A-B*K) * B);

U = K*X + F*ref;
end

== matlab function CDPR_bloques_lazo_abiertoR2020a/Controlador y Observador End Effector/MATLAB Function2 ==
  data: U input; X input; Y_err input; dX_hat output
function dX_hat = Observador(U, X, Y_err)
Kb = 1.25;
Kt = 0.516;
Jm = 0.0221;
Bm = 0.002953;
Ra = 2.581;
La = 0.0281;

a11 = -Ra/La;
a12 = -Kb/La;
a21 =  Kt/Jm;
a22 = -Bm/Jm;
b11 = 1/La;
b22 = 0;
 
A = [a11 a12; a21 a22]; 
B = [b11; b22];
C = [0 1];

Pdo = [-80 -80];

Mo1 = [C ;
      C*A];
Ho = (A-Pdo(1)*eye(2))*(A-Pdo(2)*eye(2));
L = -Ho * inv(Mo1) * [0 1].';
%Espacio de estados
dX_hat = A*X + B*U - L*Y_err;
end

== matlab function CDPR_bloques_lazo_abiertoR2020a/Planta End Effector/MATLAB Function ==
  data: U input; dX output; X input; y_acc output; Jt input
function [dX, y_acc]  = PlantaEndEffector(U, X, Jt)
b = 0.1;
m = 0.5;
g = 9.81;

A = [0 1; 
     0 -b/m]; 
 
B = [0; 
     0];

F = [0; fext];
 
dX = A*X + B*U + F ;
y_acc = dX(2);
end

== matlab function CDPR_bloques_lazo_abiertoR2020a/Controladores y observadores Motores DC [4] /Controlador y Observador Motor CD1/MATLAB Function ==
  settings: updateMethod=CONTINUOUS
  data: ref input; X input; U output
function U  = Controlador(ref, X)
Kb = 1.25;
Kt = 0.516;
Jm = 0.0221;
Bm = 0.002953;
Ra = 2.581;
La = 0.0281;

a11 = -Ra/La;
a12 = -Kb/La;
a21 =  Kt/Jm;
a22 = -Bm/Jm;
b11 = 1/La;
b22 = 0;
 
A = [a11 a12; a21 a22]; 
B = [b11; b22];
C = [Kt 0];
Pd = [-4 -4];
%Controlador
Mc = [B A*B]
H = (A-Pd(1)*eye(2))*(A-Pd(2)*eye(2));
K = -[0 1] * inv(Mc) * H;
F = 1/(C*inv(-A-B*K) * B);

U = K*X + F*ref;
end

== matlab function CDPR_bloques_lazo_abiertoR2020a/Controladores y observadores Motores DC [4] /Controlador y Observador Motor CD1/MATLAB Function2 ==
  data: U input; X input; Y_err input; dX_hat output
function dX_hat = Observador(U, X, Y_err)
Kb = 1.25;
Kt = 0.516;
Jm = 0.0221;
Bm = 0.002953;
Ra = 2.581;
La = 0.0281;

a11 = -Ra/La;
a12 = -Kb/La;
a21 =  Kt/Jm;
a22 = -Bm/Jm;
b11 = 1/La;
b22 = 0;
 
A = [a11 a12; a21 a22]; 
B = [b11; b22];
C = [0 1];

Pdo = [-80 -80];

Mo1 = [C ;
      C*A];
Ho = (A-Pdo(1)*eye(2))*(A-Pdo(2)*eye(2));
L = -Ho * inv(Mo1) * [0 1].';
%Espacio de estados
dX_hat = A*X + B*U - L*Y_err;
end

== matlab function CDPR_bloques_lazo_abiertoR2020a/Sistema de motores y carretes [4]/Sistema de motor2/Planta Motor ==
  data: U input; w_dot input; dX output; X input
function dX  = MotorCD(U, w_dot, X)
%Parametros del sistema

Kb = 1.25;
Kt = 0.516;
Jm = 0.0221;
Bm = 0.002953;
Ra = 2.581;
La = 0.0281;

a11 = -Ra/La;
a12 = -Kb/La;
a21 =  Kt/Jm;
a22 = -Bm/Jm;
b11 = 1/La;
b22 = 0;
f11 = 0;
f22 = -1/Jm;
 
A = [a11 a12; a21 a22]; 
B = [b11; b22];

F = [f11; f22];
TL = -Kt * X(1) + Jm * w_dot + Bm * X(2) ;
 
dX = A*X + B*U + F*TL;
end

== matlab function CDPR_bloques_lazo_abiertoR2020a/Planta End Effector/MATLAB Function6 ==
  settings: updateMethod=CONTINUOUS
  data: Yref output; clock input; dYref output; ddYref output
function [Yref, dYref, ddYref]  = Ref(clock)
Yref = 7*clock/15;
dYref = 7/15;
ddYref = 0;

Yref = 7 + sin(clock);
dYref = cos(clock);
ddYref = -sin(clock);
end

== matlab function CDPR_bloques_lazo_abiertoR2020a/Sistema de motores y carretes [4]/Sistema de motor3/Planta Motor ==
  data: U input; w_dot input; dX output; X input
function dX  = MotorCD(U, w_dot, X)
%Parametros del sistema

Kb = 1.25;
Kt = 0.516;
Jm = 0.0221;
Bm = 0.002953;
Ra = 2.581;
La = 0.0281;

a11 = -Ra/La;
a12 = -Kb/La;
a21 =  Kt/Jm;
a22 = -Bm/Jm;
b11 = 1/La;
b22 = 0;
f11 = 0;
f22 = -1/Jm;
 
A = [a11 a12; a21 a22]; 
B = [b11; b22];

F = [f11; f22];
TL = -Kt * X(1) + Jm * w_dot + Bm * X(2) ;
 
dX = A*X + B*U + F*TL;
end

== matlab function CDPR_bloques_lazo_abiertoR2020a/Sistema de motores y carretes [4]/Sistema de motor1/Planta Motor ==
  data: U input; w_dot input; dX output; X input
function dX  = MotorCD(U, w_dot, X)
%Parametros del sistema

Kb = 1.25;
Kt = 0.516;
Jm = 0.0221;
Bm = 0.002953;
Ra = 2.581;
La = 0.0281;

a11 = -Ra/La;
a12 = -Kb/La;
a21 =  Kt/Jm;
a22 = -Bm/Jm;
b11 = 1/La;
b22 = 0;
f11 = 0;
f22 = -1/Jm;
 
A = [a11 a12; a21 a22]; 
B = [b11; b22];

F = [f11; f22];
TL = -Kt * X(1) + Jm * w_dot + Bm * X(2) ;
 
dX = A*X + B*U + F*TL;
end

== matlab function CDPR_bloques_lazo_abiertoR2020a/Planta End Effector/MATLAB Function7 ==
  settings: updateMethod=CONTINUOUS
  data: X input; Yref input; U output; Err output; Xref output; dYref input; ddYref input
function [U, Err, Xref]  = Controlador(X, Yref, dYref, ddYref)
% Ubicación de los polos para que el error converja a cero
k1 = -4;            % Pd bloque 1
k2 = -4;            % Pd bloque 2
b2 = 1;             % valor del B(2);
b = 0.1;            % constante de friccion
m = 0.5;            % valor de la masa

% Expresion de los estados; 
x1 = X(1);
x2 = X(2);

% Ecuaciones de bloques, derivadas de los estados. 
dx1 = x2; 
%dx2 = b/m * x2 + U - 9.81;


% Ecuaciones del bloque 1
e1 = Yref - x1;                                                     % 5.4
de1 =  k1 * e1;                                                     % 5.5a
x2ref = dYref  - de1;                                               % 5.6b

% Dinamica de x3ref
dx2ref = ddYref - k1*dYref + k1*dx1;                                % 5.8

% Ecuaciones del bloque 2
e2 = x2ref - x2;                                                    % 5.9
de2 = k2*e2;                                                        % 5.10a


% Salidas del bloque, Ley de control, error y estados de referencia.
U = (1/b2)*(dx2ref +b/m * x2 - de2 + 9.81);                         % 5.16b

Err = [e1; e2];
Xref = x2ref;
end
